simulink subsystem "blood_fork"  (R2020b)
settings: Solver=VariableStepAuto  StartTime=0.0  StopTime=10.0  RelTol=1e-3
settings Model: Creator=RH  LastModifiedBy=Marco

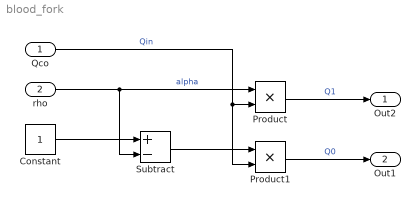
== system blood_fork ==
  Qco : Inport  Unit=liter/minute
  rho : Inport  Port=2  Unit=1
  Constant : Constant
  Product : Product
  Product1 : Product
  Subtract : Sum  Inputs=+-
  Out2 : Outport  Unit=liter/minute
  Out1 : Outport  Port=2  Unit=liter/minute
  wires:
  Product/1 -> Out2/1  "Q1"
  Qco/1 -> Product1/2, Product/2  "Qin"
  Constant/1 -> Subtract/1
  Product1/1 -> Out1/1  "Q0"
  rho/1 -> Subtract/2, Product/1  "alpha"
  Subtract/1 -> Product1/1
